simulink model "DUC_20MHZ"  (R2017b)
settings: Solver=VariableStepAuto  StartTime=0.0  StopTime=10.0  RelTol=1e-3
libraries: dspmlti4 x5
settings Model: Creator=o_cotte  LastModifiedBy=o_cotte

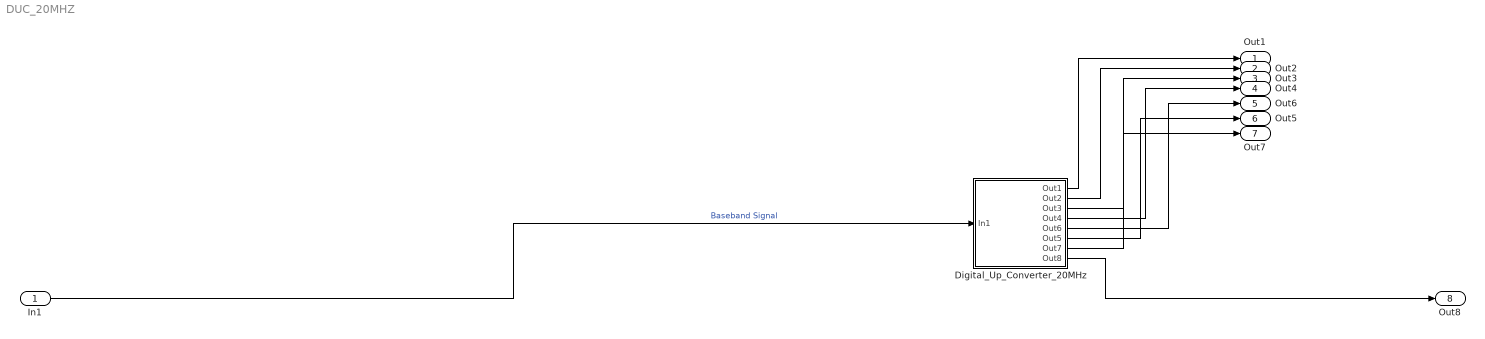
== system DUC_20MHZ ==
  In1 : Inport
  Digital_Up_Converter_20MHz : Subsystem
  Out1 : Outport
  Out2 : Outport  Port=2
  Out3 : Outport  Port=3
  Out4 : Outport  Port=4
  Out6 : Outport  Port=5
  Out5 : Outport  Port=6
  Out7 : Outport  Port=7
  Out8 : Outport  Port=8
  wires:
  In1/1 -> Digital_Up_Converter_20MHz/1(In1)  "Baseband Signal"
  Digital_Up_Converter_20MHz/1(Out1) -> Out1/1
  Digital_Up_Converter_20MHz/2(Out2) -> Out2/1
  Digital_Up_Converter_20MHz/3(Out3) -> Out3/1
  Digital_Up_Converter_20MHz/4(Out4) -> Out4/1
  Digital_Up_Converter_20MHz/5(Out6) -> Out6/1
  Digital_Up_Converter_20MHz/6(Out5) -> Out5/1
  Digital_Up_Converter_20MHz/7(Out7) -> Out7/1
  Digital_Up_Converter_20MHz/8(Out8) -> Out8/1

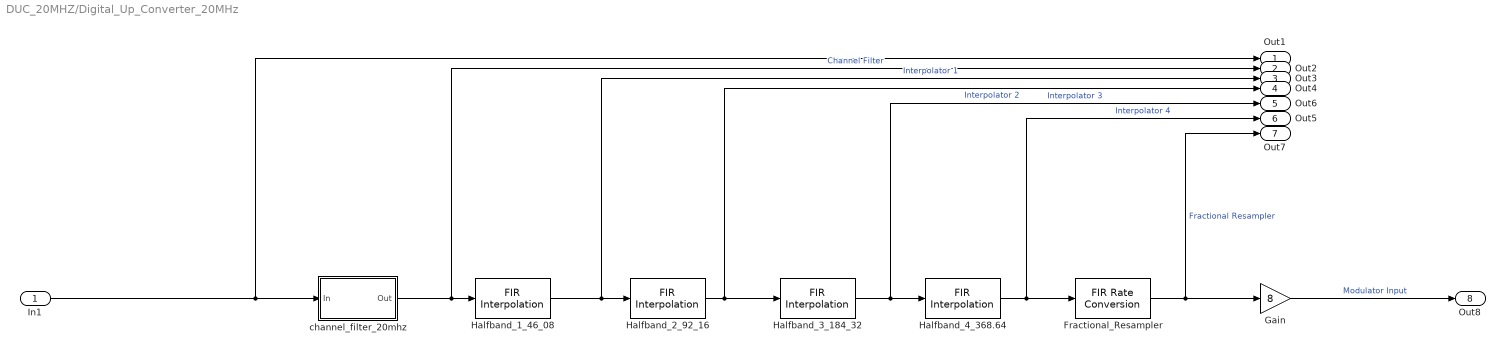
== system DUC_20MHZ/Digital_Up_Converter_20MHz ==
  In1 : Inport
  Fractional_Resampler : dspmlti4/FIR Rate Conversion  Tag=BlockMethodSubSystem  FilterSource=Dialog parameters  L=4  h=[-0.000847148666357944776 -0.00411604851397991828 -0.0104519083418887458 -0.0161494458717064242 -0.0113821512901921551 0.0159050187160891913 0.0704610974207035695 0.141170423824235752 0.202248552859676994 0.226490421520463531 0.202248552859676994 0.141170423824235752 0.0704610974207035695 0.0159050187160891913 -0.0113821512901921551 -0.0161494458717064242 -0.0104519083418887458 -0.00411604851397991828 -0.000847148666357944776]  M=3  FilterObject=FRC  roundingMode=Floor  overflowMode=off  firstCoeffDataTypeStr=Inherit: Same word length as input  firstCoeffMin=[]  firstCoeffMax=[]  firstCoeffLastDataTypeStr=Inherit: Same word length as input  outputDataTypeStr=Inherit: Same as accumulator  outputMin=[]  outputMax=[]  outputLastDataTypeStr=Inherit: Same as accumulator
      settings: SourceProductName=DSP System Toolbox  SourceProductBaseCode=DS
  Gain : Gain  Gain=8
  Halfband_1_46_08 : dspmlti4/FIR Interpolation  Tag=BlockMethodSubSystem  FilterSource=Dialog parameters  h=[0.00766036227638032356 0 -0.0536604116251646474 0 0.296025845822847244 0.5 0.296025845822847244 0 -0.0536604116251646474 0 0.00766036227638032356]  L=2  FilterObject=FINTERP  framing=Allow multirate processing  outputBufInitCond=0  roundingMode=Floor  overflowMode=off  firstCoeffDataTypeStr=Inherit: Same word length as input  firstCoeffMin=[]  firstCoeffMax=[]  firstCoeffLastDataTypeStr=Inherit: Same word length as input  outputDataTypeStr=Inherit: Same as accumulator  outputMin=[]  outputMax=[]  outputLastDataTypeStr=Inherit: Same as accumulator
      settings: SourceProductName=DSP System Toolbox
  Halfband_2_92_16 : dspmlti4/FIR Interpolation  Tag=BlockMethodSubSystem  FilterSource=Dialog parameters  h=[0.00766036227638032356 0 -0.0536604116251646474 0 0.296025845822847244 0.5 0.296025845822847244 0 -0.0536604116251646474 0 0.00766036227638032356]  L=2  FilterObject=FINTERP  framing=Allow multirate processing  outputBufInitCond=0  roundingMode=Floor  overflowMode=off  firstCoeffDataTypeStr=Inherit: Same word length as input  firstCoeffMin=[]  firstCoeffMax=[]  firstCoeffLastDataTypeStr=Inherit: Same word length as input  outputDataTypeStr=Inherit: Same as accumulator  outputMin=[]  outputMax=[]  outputLastDataTypeStr=Inherit: Same as accumulator
      settings: SourceProductName=DSP System Toolbox
  Halfband_3_184_32 : dspmlti4/FIR Interpolation  Tag=BlockMethodSubSystem  FilterSource=Dialog parameters  h=[-0.0325201718357778641 0 0.28248678153183715 0.5 0.28248678153183715 0 -0.0325201718357778641]  L=2  FilterObject=FINTERP  framing=Allow multirate processing  outputBufInitCond=0  roundingMode=Floor  overflowMode=off  firstCoeffDataTypeStr=Inherit: Same word length as input  firstCoeffMin=[]  firstCoeffMax=[]  firstCoeffLastDataTypeStr=Inherit: Same word length as input  outputDataTypeStr=Inherit: Same as accumulator  outputMin=[]  outputMax=[]  outputLastDataTypeStr=Inherit: Same as accumulator
      settings: SourceProductName=DSP System Toolbox
  Halfband_4_368.64 : dspmlti4/FIR Interpolation  Tag=BlockMethodSubSystem  FilterSource=Dialog parameters  h=[-0.0315620277130336316 0 0.281559967967666802 0.5 0.281559967967666802 0 -0.0315620277130336316]  L=2  FilterObject=FINTERP  framing=Allow multirate processing  outputBufInitCond=0  roundingMode=Floor  overflowMode=off  firstCoeffDataTypeStr=Inherit: Same word length as input  firstCoeffMin=[]  firstCoeffMax=[]  firstCoeffLastDataTypeStr=Inherit: Same word length as input  outputDataTypeStr=Inherit: Same as accumulator  outputMin=[]  outputMax=[]  outputLastDataTypeStr=Inherit: Same as accumulator
      settings: SourceProductName=DSP System Toolbox
  channel_filter_20mhz : Subsystem  Tag=BlockMethodSubSystem
  Out1 : Outport
  Out2 : Outport  Port=2
  Out3 : Outport  Port=3
  Out4 : Outport  Port=4
  Out6 : Outport  Port=5
  Out5 : Outport  Port=6
  Out7 : Outport  Port=7
  Out8 : Outport  Port=8
  wires:
  Halfband_1_46_08/1 -> Out3/1, Halfband_2_92_16/1  "Interpolator 1"
  Halfband_4_368.64/1 -> Out5/1, Fractional_Resampler/1  "Interpolator 4"
  Halfband_3_184_32/1 -> Out6/1, Halfband_4_368.64/1  "Interpolator 3"
  Gain/1 -> Out8/1  "Modulator Input"
  Fractional_Resampler/1 -> Out7/1, Gain/1  "Fractional Resampler"
  Halfband_2_92_16/1 -> Out4/1, Halfband_3_184_32/1  "Interpolator 2"
  channel_filter_20mhz/1(Out) -> Out2/1, Halfband_1_46_08/1  "Channel Filter"
  In1/1 -> Out1/1, channel_filter_20mhz/1(In)

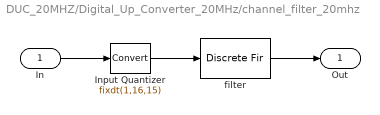
== system DUC_20MHZ/Digital_Up_Converter_20MHz/channel_filter_20mhz ==
  In : Inport
  Input Quantizer : DataTypeConversion  OutDataTypeStr=fixdt(1,16,15)  RndMeth=Round  SaturateOnIntegerOverflow=on
  filter : DiscreteFir  Coefficients=[0.00196720306212561482 0.00149425216106443691 -0.00400293320810243911 0.00390100375479263085 -2.89147778793418149e-07 -0.00382987035567847927 0.00259524746093026722 0.00299398664123881825 -0.00593452115673513431 0.00124990544593627895 0.00637795842127835896 -0.00686348731071946636 -0.00221497240802292442 0.0103098487689475479 -0.00579957522561930575 -0.00783937474606764828 0.0135158399775277549 -0.00155602281125578911 -0.0151258138642529176 0.0142568491821450007 0.00665092392134642753 -0.0226731257471077807 0.0104679129061562917 0.018904809782294061 -0.0281519456111425509 3.77195008409268937e-05 0.0343690574379760388 -0.0283201893723893684 -0.0191525533345231584 0.0512858826615412086 -0.0186277130508248137 -0.0502110306645960694 0.0672661641118006554 0.00945698178191303231 -0.102591535984214791 0.0797527182394069389 0.0877414496207477579 -0.237055871068311774 0.0866069815926385905 1 1 0.0866069815926385905 -0.237055871068311774 0.0877414496207477579 0.0797527182394069389 -0.102591535984214791 0.00945698178191303231 0.0672661641118006554 -0.0502110306645960694 -0.0186277130508248137 0.0512858826615412086 -0.0191525533345231584 -0.0283201893723893684 0.0343690574379760388 3.77195008409268937e-05 -0.0281519456111425509 0.018904809782294061 0.0104679129061562917 -0.0226731257471077807 0.00665092392134642753 0.0142568491821450007 -0.0151258138642529176 -0.00155602281125578911 0.0135158399775277549 -0.00783937474606764828 -0.00579957522561930575 0.0103098487689475479 -0.00221497240802292442 -0.00686348731071946636 0.00637795842127835896 0.00124990544593627895 -0.00593452115673513431 0.00299398664123881825 0.00259524746093026722 -0.00382987035567847927 -2.89147778793418149e-07 0.00390100375479263085 -0.00400293320810243911 0.00149425216106443691 0.00196720306212561482]  CoefDataTypeStr=fixdt(true,16,14)  ProductDataTypeStr=fixdt(true,31,30)  AccumDataTypeStr=fixdt(true,33,30)  OutDataTypeStr=fixdt(true,33,30)  RndMeth=Ceiling  SaturateOnIntegerOverflow=on
  Out : Outport
  wires:
  In/1 -> Input Quantizer/1
  Input Quantizer/1 -> filter/1
  filter/1 -> Out/1
